simulink model "GEB_ASHP"  (R2020a)
settings: Solver=FixedStepAuto  StartTime=15*24*3600  StopTime=15*24*3600+30*60  FixedStep=60  RelTol=1e-5
undefined symbols (not defined in the file or in its folder): Discrete, Time
libraries: ctrlSharedLib x1
settings Model: Creator=zhelu  LastModifiedBy=yl3328

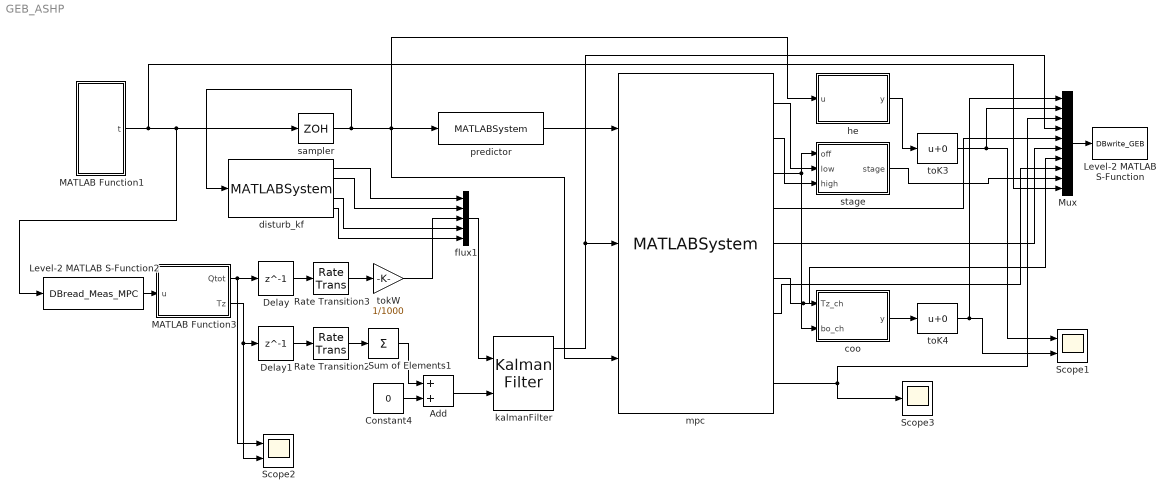
== system GEB_ASHP ==
  Add : Sum
  Constant4 : Constant  Value=0
  Delay : Delay  DelayLength=1  SampleTime=60
  Delay1 : Delay  DelayLength=1  InitialCondition=20  SampleTime=60
  Level-2 MATLAB S-Function : M-S-Function  FunctionName=DBwrite_GEB
  Level-2 MATLAB S-Function2 : M-S-Function  FunctionName=DBread_Meas_MPC
  MATLAB Function1 : MATLAB Function  TreatAsAtomicUnit=on
  MATLAB Function3 : MATLAB Function  TreatAsAtomicUnit=on
  Mux : Mux  Inputs=10
  Rate Transition2 : RateTransition  OutPortSampleTime=900
  Rate Transition3 : RateTransition  OutPortSampleTime=900
  Scope1 : Scope  NumInputPorts=2
  Scope2 : Scope  NumInputPorts=2
  Scope3 : Scope
  Sum of Elements1 : Sum  Inputs=+
  coo : MATLAB Function  TreatAsAtomicUnit=on
  disturb_kf : MATLABSystem  System=get_predictors_block_kalman  PH=1  CH=1  dt=900  np=5  SimulateUsing=Interpreted execution
      mask Type: get_predictors_block_kalman
      mask Display:
      | disp('get_predictors_block_kalman');
      | port_label('input',1,'time');
      | port_label('output',1,'out1');
      | port_label('output',2,'out2');
      | port_label('output',3,'out3');
      | port_label('output',4,'out4');
      | port_label('output',5,'out5');
  flux1 : Concatenate  NumInputs=5
  he : MATLAB Function  TreatAsAtomicUnit=on
  kalmanFilter : ctrlSharedLib/Kalman Filter  TimeDomain=Discrete-Time  UseCurrentEstimator=on  ModelSource=Individual A, B, C, D matrices  ModelSourceVariable=ss(0.95,1,1,0,1)  A=[0.863099253142606,0,0.109354030032509;0,0.990777163068422,0.001620677259379;0.014228034719401,0.002160031123503,0.983611934157095]  B=[0.0275,0.1844,0.1844,0,0;0.0076,0,0,0.0180,0;0,0,0,0,0.0240]  C=[1,0,0]  D=0  NumberOfStates=1  NumberOfInputs=1  NumberOfOutputs=1  InitialEstimateSource=Dialog  X0=[27.1006, 1.2071, -239.2718]  P0=10  UseK=off  UseGH=off  NumberOfProcessNoiseInputs=1  G=[1,0;0,1;1,0;0,1]  TimeInvariantG=on  H=0  TimeInvariantH=on  Q=diag([1, 1, 1])  TimeInvariantQ=on  R=0.5  TimeInvariantR=on  N=0  TimeInvariantN=on  AddInputPort=on  AddEnablePort=off  OutputEstimatedY=on  OutputP=on  Ts=-1
  mpc : MATLABSystem  System=mpc_cooling_milp  PH=1  CH=1  dt=900  q_cl_min=0  q_cl_max=100  q_ch_min=0  q_ch_max=100  p_cl_min=0  p_cl_max=100  p_ch_min=0  p_ch_max=100  occ_start=6  occ_end=22  nu=8  w=[ 1, 1000, 0 ]  u_lb=[ 0, 0, 0, 0, 0, 0, 0, 0 ]  u_ub=[ 1, 1, 1, 20, 20, 100, 100, 0.1 ]  price_tou="[0.00746     0.00746     0.00746     0.00746     0.00746     0.00746     0.00746     0.00746     0.00746     0.00746     0.00746     0.00746     0.00746     0.01692     0.01692     0.01692     0.01692     0.01692     0.00746     0.00746     0.00746     0.00746     0.00746     0.00746]"  SimulateUsing=Interpreted execution
      mask Type: mpc_cooling_milp
      mask Display:
      | disp('mpc_cooling_milp');
      | port_label('input',1,'predictor');
      | port_label('input',2,'states');
      | port_label('input',3,'time');
      | port_label('output',1,'b_cl_ch');
      | port_label('output',2,'b_ch_ch');
      | port_label('output',3,'bo_ch');
      | port_label('output',4,'p_pred_ch');
      | port_label('output',5,'q_pred_ch');
      | port_label('output',6,'Tz_pred_ch');
      | port_label('output',7,'price_ch');
      | port_label('output',8,'nOpt_steps');
      | port_label('output',9,'optimalFlag');
  predictor : MATLABSystem  System=get_predictors_block_15min  PH=1  CH=1  dt=900  np=5  SimulateUsing=Interpreted execution
      mask Type: get_predictors_block_15min
      mask Display:
      | disp('get_predictors_block_15min');
      | port_label('input',1,'time');
      | port_label('output',1,'predictors');
  sampler : ZeroOrderHold  SampleTime=900
  stage : MATLAB Function  TreatAsAtomicUnit=on
  toK3 : Bias
  toK4 : Bias
  tokW : Gain  Gain=1/1000
  wires:
  Rate Transition3/1 -> tokW/1
  Constant4/1 -> Add/2
  Rate Transition2/1 -> Sum of Elements1/1
  coo/1(y) -> toK4/1
  disturb_kf/2 -> flux1/2
  kalmanFilter/1 -> Mux/4, mpc/2
  disturb_kf/4 -> flux1/4
  mpc/3 -> coo/2(bo_ch), stage/1(off)
  disturb_kf/1 -> flux1/1
  MATLAB Function3/1(Qtot) -> Scope2/1, Delay/1
  MATLAB Function3/2(Tz) -> Scope2/2, Delay1/1
  Delay1/1 -> Rate Transition2/1
  sampler/1 -> he/1(u), mpc/3, predictor/1, disturb_kf/1
  disturb_kf/5 -> flux1/5
  Add/1 -> kalmanFilter/2
  mpc/6 -> Mux/7, coo/1(Tz_ch)
  predictor/1 -> mpc/1
  Sum of Elements1/1 -> Add/1
  he/1(y) -> toK3/1
  flux1/1 -> kalmanFilter/1
  Delay/1 -> Rate Transition3/1
  tokW/1 -> flux1/3
  Level-2 MATLAB S-Function2/1 -> MATLAB Function3/1(u)
  MATLAB Function1/1(t) -> Mux/10, Level-2 MATLAB S-Function2/1, sampler/1
  toK3/1 -> Mux/2, Scope1/1
  toK4/1 -> Mux/1, Scope1/2
  Mux/1 -> Level-2 MATLAB S-Function/1
  mpc/9 -> Scope3/1, Mux/3
  mpc/4 -> Mux/5
  mpc/5 -> Mux/6
  mpc/7 -> Mux/8
  mpc/1 -> stage/2(low)
  mpc/2 -> stage/3(high)
  stage/1(stage) -> Mux/9

== matlab function GEB_ASHP/stage ==
  data: off input; low input; stage output; high input
function stage = fcn(off,low,high)
% detemine the stage of MPC predict
[a,b]=max([off,low,high]);
stage=b-1;

== matlab function GEB_ASHP/coo ==
  data: Tz_ch input; y output; bo_ch input
function y = fcn(Tz_ch, bo_ch)
% transfer predicted zone temperature to heating setpoint
% - when heating is off, the zone temperature setpoint is set to heating
% lower bound so that local heat pump controller wont activate heating
% - when heating is on, the predicted zone temperature is treated as zone
% temperature setpoint
% -------------------------------------------------
TCooHig = 30;

% off 
if bo_ch > 0
    y = TCooHig;
else % on
    y = Tz_ch;
end

== matlab function GEB_ASHP/he ==
  data: u input; y output
function y = fcn(u)
% to control horizon signal
THea = 20*ones(1, 24);
THea(8:18) = 20;
h = floor(mod(u, 86400)/3600) + 1;
y = THea(h);

== matlab function GEB_ASHP/MATLAB Function1 ==
  data: t output
function t  = fcn
coder.extrinsic('xlsread');
T=0;
[T] = xlsread('Time.xlsx', 1,'B1');
t=0;
t=T+15*60; %237*86400+645*60;

== matlab function GEB_ASHP/MATLAB Function3 ==
  data: Qtot output; u input; Tz output
function [Qtot,Tz] = fcn(u)
%% Inputs
% Tin:  inlet air temperature [°C]
% Tout: outlet air temperature [°C]
% win:  inlet air humidity ratio [kg/kg]
% wout: outlet air humidity ratio [kg/kg]
% m:    inlet air mass flow rate [kg/s]
%% Outputs
% Qtot: total load [W]
% Tz: Tz = Tout, zone air temperature [°C]
%% Main
% initialization
Tin = zeros(1);
Tout = zeros(1);
win = zeros(1);
wout = zeros(1);
m = zeros(1);
% inputs
Tin = u(1);
Tout = u(2);
win = u(3);
wout = u(4);
m = u(5);
% properties
cpa = 1.006;
cpw = 1.86;
hwe = 2501;
% enthalpy
hin = cpa*Tin + win.*(cpw*Tin + hwe);
hout = cpa*Tout + wout.*(cpw*Tout + hwe);
% outputs
Qtot = 1000*m.*(hin - hout);
Tz = Tout;
